simulink model "kite"  (R2022b)
settings: Solver=VariableStepAuto  StartTime=0.0  StopTime=t_sim  FixedStep=stepSize  MinStep=1e-3  RelTol=1e-3
values from neighbouring files (symbols this model uses):
  V_WR = 30/3.6    (= 8.33333333333)    [Init_sim.m]
  x0 = [theta_0; phi_0; dtheta_0; dphi_0; psi_0]    [Init_sim.m]
undefined symbols (not defined in the file or in its folder): params
settings Model: Creator=Louis  LastModifiedBy=LouisCassany
settings SolverCC: MaxConsecutiveMinStep=10  AlgebraicLoopSolver=TrustRegion
settings DataIOCC: SaveState=on
settings DebuggingCC: UnconnectedInputMsg=warning  UnconnectedOutputMsg=warning  UnconnectedLineMsg=warning  SFMachineParentedDataDiag=warning  ArithmeticOperatorsInVariantConditions=warning
settings ModelReferenceCC: EnableRefExpFcnMdlSchedulingChecks=on
settings SFSimCC: CustomCodeUndefinedFunction=UseInterfaceOnly

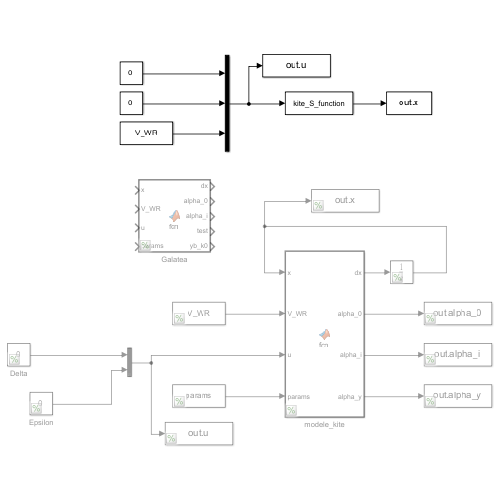
[thumbnail: Simulink's stored preview of the top-level diagram]
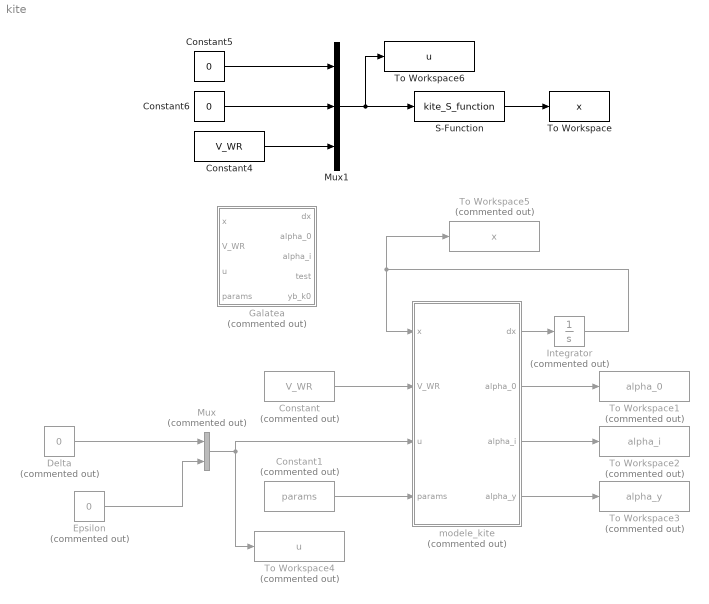
== system kite ==
  Constant : Constant  Commented=on  Value=V_WR
  Constant1 : Constant  Commented=on  Value=params
  Constant4 : Constant  Value=V_WR
  Constant5 : Constant  Value=0
  Constant6 : Constant  Value=0
  Delta : Constant  Commented=on  Value=0
  Epsilon : Constant  Commented=on  Value=0
  Galatea : MATLAB Function  Commented=on  TreatAsAtomicUnit=on
  Integrator : Integrator  Commented=on  InitialCondition=x0
  Mux : Mux  Commented=on  Inputs=2
  Mux1 : Mux  Inputs=3
  S-Function : S-Function  FunctionName=kite_S_function  Parameters=x0  SFunctionDeploymentMode=off  EnableBusSupport=off
  To Workspace : ToWorkspace  VariableName=x  SaveFormat=Timeseries  SampleTime=-1
  To Workspace1 : ToWorkspace  Commented=on  VariableName=alpha_0  SaveFormat=Timeseries  SampleTime=-1
  To Workspace2 : ToWorkspace  Commented=on  VariableName=alpha_i  SaveFormat=Timeseries  SampleTime=-1
  To Workspace3 : ToWorkspace  Commented=on  VariableName=alpha_y  SaveFormat=Timeseries  SampleTime=-1
  To Workspace4 : ToWorkspace  Commented=on  VariableName=u  SaveFormat=Timeseries  SampleTime=-1
  To Workspace5 : ToWorkspace  Commented=on  VariableName=x  SaveFormat=Timeseries  SampleTime=-1
  To Workspace6 : ToWorkspace  VariableName=u  SaveFormat=Timeseries  SampleTime=-1
  "modele_kite " : MATLAB Function  Commented=on  TreatAsAtomicUnit=on
  wires:
  "modele_kite "/2(alpha_0) -> To Workspace1/1
  "modele_kite "/3(alpha_i) -> To Workspace2/1
  "modele_kite "/1(dx) -> Integrator/1
  Constant1/1 -> "modele_kite "/4(params)
  "modele_kite "/4(alpha_y) -> To Workspace3/1
  Integrator/1 -> To Workspace5/1, "modele_kite "/1(x)
  Constant/1 -> "modele_kite "/2(V_WR)
  Mux/1 -> "modele_kite "/3(u), To Workspace4/1
  Delta/1 -> Mux/1
  Epsilon/1 -> Mux/2
  Mux1/1 -> To Workspace6/1, S-Function/1
  Constant4/1 -> Mux1/3
  Constant5/1 -> Mux1/1
  S-Function/1 -> To Workspace/1
  Constant6/1 -> Mux1/2

== matlab function kite/modele_kite  ==
  data: x input; V_WR input; u input; dx output; alpha_0 output; params input; alpha_i output; alpha_y output
function [dx, alpha_0, alpha_i, alpha_y] = fcn(x, V_WR, u, params)

% Constant parameters
r = params(1);
m = params(2);
g_k = params(3);
M_k = params(4);
A_k = params(5);
rho_air = params(6);
g = params(7);
K_i = params(8);
alpha_i0 = params(9);
C_D = params(10);
C_L = params(11);
C_T = params(12);

% Transformation matrices
Mx = @(alpha) [1 0 0; 0 cos(alpha) sin(alpha); 0 -sin(alpha) cos(alpha)];
My = @(alpha) [cos(alpha) 0 sin(alpha); 0 1 0; -sin(alpha) 0 cos(alpha)];
Mz = @(alpha) [cos(alpha) -sin(alpha) 0; sin(alpha) cos(alpha) 0; 0 0 1];

%%
phi = x(1);
theta = x(2);
dphi = x(3);
dtheta = x(4);
psi = x(5);

delta = u(1);
epsilon = u(2);

WR_M_k0 = Mz(phi)*My(theta-pi/2); % from Rk0 to RWR
V_WR = [V_WR;0;0];
V_k_k0 = [-r*dtheta;r*dphi*cos(theta);0]; % Kite's speed in Rk0
V_a_WR = V_WR-WR_M_k0*V_k_k0;
modV_a = norm(V_a_WR);

k0_M_b = Mz(pi+psi);
xb_k0 = k0_M_b*[1;0;0];
yb_k0 = k0_M_b*[0;1;0];
zb_k0 = k0_M_b*[0;0;1];
xa_WR = -V_a_WR/modV_a;
xa_k0 = WR_M_k0.'*xa_WR;

%%

alpha_0 = pi/2 - acos(dot(zb_k0,xa_k0)/(norm(zb_k0)*norm(xa_k0)));
alpha_i = K_i*epsilon+alpha_i0;
alpha = alpha_0 + alpha_i;

x_ap_k0 = [xa_k0(1);xa_k0(2);0]/norm([xa_k0(1);xa_k0(2);0]);

C = dot(x_ap_k0,xb_k0)/(norm(dot(x_ap_k0,xb_k0)));
S = (xb_k0(1)*x_ap_k0(2)-xb_k0(2)*x_ap_k0(1));
alpha_y = real(sign(S)*acos(C));

lift = 0.5*rho_air*C_L*alpha*A_k*modV_a*modV_a;
drag = 0.5*rho_air*C_D*alpha*A_k*modV_a*modV_a;
trans = 0.5*rho_air*C_T*alpha_y*A_k*modV_a*modV_a;


x_lift_k0=cross(-xa_k0,yb_k0)/norm(cross(-xa_k0,yb_k0));
x_drag_k0= -xa_k0;

F_a_k0 = lift*(x_lift_k0)+drag*(x_drag_k0)+trans*(-yb_k0);

P_k0 = [m*g*cos(theta); 0; m*g*sin(theta)];

F_ext_k0 = P_k0 + F_a_k0;

V_a_Rb=k0_M_b'*WR_M_k0'*V_a_WR;
va = -V_a_Rb(1);

ddtheta = (-F_ext_k0(1)/(r*m))-sin(theta)*cos(theta)*dphi^2;
ddphi = (F_ext_k0(2)/(r*m*cos(theta)))+ 2*tan(theta)*dtheta*dphi;
dpsi = g_k*va*delta+(M_k*((cos(theta)*sin(psi))/va))-dphi*sin(theta);

dx = [dphi; dtheta; ddphi; ddtheta; dpsi];

end

== matlab function kite/Galatea ==
  data: x input; V_WR input; u input; dx output; params input; alpha_0 output; alpha_i output; test output; yb_k0 output
function [dx, alpha_0, alpha_i,test,yb_k0]  = fcn(x, V_WR, u, params)

%% Constant parameters
r = params(1);
m = params(2);
g_k = params(3);
M_k = params(4);
A_k = params(5);
rho_air = params(6);
g = params(7);
K_i = params(8);
alpha_i0 = params(9);
C_D = params(10);
C_L = params(11);
C_T = params(12);

%% State
phi = x(1);
theta = x(2);
dphi = x(3);
dtheta = x(4);
psi = x(5);

omega_theta = dtheta; 
omega_phi = dphi;

%% Inputs
delta = u(1);
epsilon = u(2);
yb_k0 = [sin(psi);-cos(psi);0];

%% Dynamics
V_k_2 = r^2*(omega_theta^2+omega_phi^2*cos(theta)^2);
test=sqrt(V_k_2);
V_a = sqrt(V_k_2+V_WR^2+2*r*V_WR*(cos(phi)*sin(theta)*omega_theta+sin(phi)*cos(theta)*omega_phi));
alpha_0 = asin(cos(phi)*cos(theta)*V_WR/V_a);
alpha_i = K_i*epsilon + alpha_i0;
alpha = alpha_0 + alpha_i;
A_DL = (rho_air*A_k*V_a^2)/(2*m*r)*(cos(alpha_0)*C_D*alpha-sin(alpha_0)*C_L*alpha);

domega_phi = 2*tan(theta)*omega_phi*omega_theta+sin(psi)/cos(theta)*A_DL;
domega_theta = -sin(theta)*cos(theta)*omega_phi^2-cos(psi)*A_DL-(g*cos(theta))/(r);
dpsi = g_k*cos(alpha)*V_a*delta+M_k*(cos(theta)*sin(psi))/(cos(alpha)*V_a)-omega_phi*sin(theta);

dx=[omega_phi; omega_theta; domega_phi; domega_theta; dpsi];
